simulink model "Week3Problem1"  (R2020b)
settings: Solver=VariableStepAuto  StartTime=0.0  StopTime=10.0  RelTol=1e-3
settings Model: Creator=HP  LastModifiedBy=HP

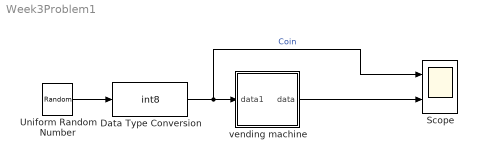
== system Week3Problem1 ==
  Data Type Conversion : DataTypeConversion  OutDataTypeStr=int8  RndMeth=Nearest  SaturateOnIntegerOverflow=on
  Scope : Scope  NumInputPorts=2
  Uniform Random Number : UniformRandomNumber  Minimum=0  Maximum=2  Seed=337  SampleTime=10
  vending machine : Stateflow chart  TreatAsAtomicUnit=on
  wires:
  Uniform Random Number/1 -> Data Type Conversion/1
  Data Type Conversion/1 -> vending machine/1(data1), Scope/1  "Coin"
  vending machine/1(data) -> Scope/2

== stateflow chart Week3Problem1/vending machine ==
  settings: stateMachineType=MEALY_MACHINE
  state Got_0
  state Got_Nickel
  state Got_Dime
  (default) -> Got_0
  Got_0 -> Got_Nickel [order 1] : [data1==1]{data=0}
  Got_Nickel -> Got_0 [order 1] : [data1==2]{data=1}
  Got_Dime -> Got_0 [order 2] : [data1==1]{data=1}
  Got_0 -> Got_Dime [order 2] : [data1==2]{data=0}
  Got_Nickel -> Got_Dime [order 2] : [data1==1]{data=0}
  Got_Dime -> Got_Nickel [order 1] : [data1==2]{data=1}
  data: data output; data1 input
